simulink model "SPM_PSO"  (R2025a)
settings: Solver=VariableStepAuto  StartTime=0.0  StopTime=50000  RelTol=1e-3  AbsTol=1e-3  EnableMultiTasking=on
model workspace (MAT data in the model file):
  I = 6.58273420006
  I1 = 7.80289756193
  I2 = 6.88130880881
  SOC_break = 0.782129341538
libraries: fl_lib x8, nesl_utility x4, BatteryCurrentManagement x1, batt_lib x1, simulink x1, BatteryEstimators x1
settings Model: Creator=praji  LastModifiedBy=praji
settings SolverCC: AutoScaleAbsTol=off  AlgebraicLoopSolver=TrustRegion  MaxZcPerStep=1.0
settings DataIOCC: LimitDataPoints=on  MaxDataPoints=10000
settings OptimizationCC: ReuseModelBlockBuffer=off  LifeSpan=inf
settings DebuggingCC: UnconnectedInputMsg=warning  UnconnectedOutputMsg=warning  UnconnectedLineMsg=warning  AllowSymbolicDim=off  SFUnexpectedBacktrackingDiag=warning  SFNoUnconditionalDefaultTransitionDiag=warning  SFExecutionAtInitializationDiag=none  ArithmeticOperatorsInVariantConditions=warning
settings ModelReferenceCC: EnableRefExpFcnMdlSchedulingChecks=on
settings SFSimCC: SimUseLocalCustomCode=off  CustomCodeUndefinedFunction=UseInterfaceOnly
settings RTWCC: RTWUseLocalCustomCode=off  GPUComputeCapability=3.5  DLArmComputeVersion=19.05
settings CodeAppCC: StateflowObjectComments=on
settings GRTTargetCC: TargetLangStandard=C89/C90 (ANSI)
settings ConfigComp: CovMetricSettings=dw  CovSaveCumulativeToWorkspaceVar=on  CovSaveSingleToWorkspaceVar=on  CovExternalEMLEnable=off  CovSFcnEnable=off
settings SimscapeCC: SimscapeLogType=all  SimscapeLogSimulationStatistics=on  SimscapeLogDataHistory=10000.0

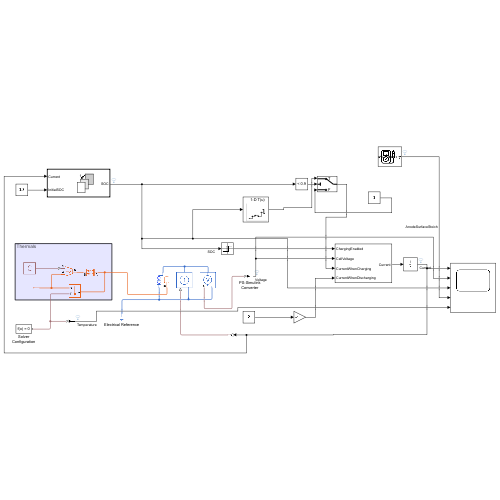
[thumbnail: Simulink's stored preview of the top-level diagram]
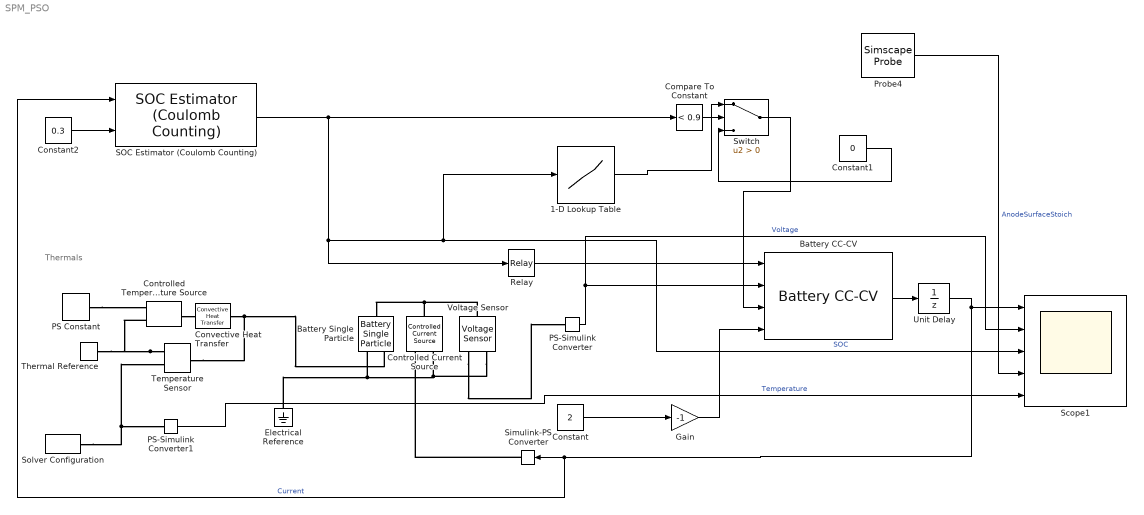
== system SPM_PSO ==
  note: Thermals
  1-D Lookup Table : Lookup_n-D  NumberOfTableDimensions=1  BreakpointsForDimension1=[0 SOC_break 1]  Table=[I1 I2 I2]  InterpMethod=Flat  InternalRulePriority=Speed  RndMeth=Simplest
  Battery CC-CV : BatteryCurrentManagement/Battery CC-CV  MinMaxFlag=off  MaxCellVoltage=3.65  Kp=100  Ki=10  Kaw=1  Kt=1  Ts=1
      settings: LibrarySourceBlock=batt_sl_lib/Current Management/Battery CC-CV
  Battery Single Particle : batt_lib/Cells/Electrochemical/Battery Single Particle  ExtrapolationMethod=simscape.enum.extrapolation.nearest  ThicknessAnode=8.52e-5 m  ElectrolyteLayerCountAnode=10  ThicknessSeparator=1.20e-5 m  ElectrolyteLayerCountSeparator=5  ThicknessCathode=7.56e-5 m  ElectrolyteLayerCountCathode=10  ElectrodePlateArea=0.177 m^2  ParticleRadiusAnode=5.86e-6 m  ShellCountAnode=20  ParticleRadiusCathode=5.22e-6 m  ShellCountCathode=25  ActiveMaterialVolumeFractionAnode=0.75  ActiveMaterialVolumeFractionCathode=0.665  StoichiometryBreakpointsSpecification=simscape.battery.enum.cells.electrochemical.StoichiometryBreakpointsSpecification.absolute  NormalizedStoichiometryBreakpoints=linspace(0.01, 0.90, 39)  OpenCircuitPotentialAnode=|  OpenCircuitPotentialCathode=|  AbsoluteStoichiometryBreakpointsAnode=linspace(0.01, 0.90, 39)  OpenCircuitPotentialAbsoluteAnode=[.484; .335; .253; .209; .2; .181; .165; .151; .139; .131; .128; .125; .124; .124; .123; .122; .119; .117; .111; .108; .101; .098; .095; .093; .092; .088; .088; .088; .088; .087; .087; .087; .085; .082; .079; .071; .064; .049; .026] V  AbsoluteStoichiometryBreakpointsCathode=linspace(0.02, 0.95, 39)  OpenCircuitPotentialAbsoluteCathode=[3.81; 3.608; 3.512; 3.478; 3.459; 3.453; 3.45257; 3.45214; 3.45171; 3.45128; 3.45085; 3.45042; 3.44999; 3.44956; 3.44913; 3.4487; 3.44827; 3.44784; 3.44741; 3.44698; 3.44655; 3.44612; 3.44569; 3.44526; 3.44483; 3.4444; 3.44397; 3.44354; 3.44311; 3.44268; 3.44225; 3.44182; 3.44139; 3.44096; 3.44053; 3.44; 3.412; 3.304; 2.968] V  MaximumConcentrationAnode=33133 mol/m^3  MaximumStoichiometryAnode=0.90  MinimumStoichiometryAnode=0.01  MaximumConcentrationCathode=63104 mol/m^3  MaximumStoichiometryCathode=0.95  MinimumStoichiometryCathode=0.02  ActiveMaterialDiffusionCoefficientAnode=3.3E-14 m^2/s  ActiveMaterialDiffusionCoefficientCathode=4E-15 m^2/s  ConductivityAnode=100 S/m  ConductivityCathode=10 S/m  CurrentCollectorResistance=0 Ohm  ElectrolyteVolumeFractionAnode=0.25  ElectrolyteVolumeFractionSeparator=0.45  ElectrolyteVolumeFractionCathode=0.335  ElectrolyteConductivity=0.29 S/m  BruggemanExponentAnode=1.5  BruggemanExponentSeparator=1.5  BruggemanExponentCathode=1.5  TransferenceNumber=0.2594  ElectrolyteDiffusionCoefficient=2.6E-10 m^2/s  ChargeTransferRateAnode=6.48e-7 m^(5/2)/(mol^(1/2)*s)  ChargeTransferRateCathode=3.42e-6 m^(5/2)/(mol^(1/2)*s)  BatteryThermalMass=50 J/K  ArrheniusReferenceTemperature=298.15 K  ActiveMaterialDiffusionActivationEnergyAnode=35000 J/mol  ActiveMaterialDiffusionActivationEnergyCathode=35000 J/mol  ElectrolyteDiffusionActivationEnergy=26600 J/mol  ConductivityActivationEnergyAnode=3000 J/mol  ConductivityActivationEnergyCathode=3000 J/mol  ElectrolyteConductivityActivationEnergy=11000 J/mol  ChargeTransferActivationEnergyAnode=35000 J/mol  ChargeTransferActivationEnergyCathode=17800 J/mol  batteryCurrent_specify=off  batteryCurrent_priority=None  batteryCurrent=0 A  batteryCurrent_nominal_specify=off  batteryCurrent_nominal_value=1  batteryCurrent_nominal_unit=A  batteryVoltage_specify=off  batteryVoltage_priority=High  batteryVoltage=3.65 V  batteryVoltage_nominal_specify=on  batteryVoltage_nominal_value=3.65  batteryVoltage_nominal_unit=V  averageElectrolyteConcentration_specify=off  averageElectrolyteConcentration_priority=High  averageElectrolyteConcentration=1200 mol/m^3  averageElectrolyteConcentration_nominal_specify=off  averageElectrolyteConcentration_nominal_value=1  averageElectrolyteConcentration_nominal_unit=mol/m^3  stateOfCharge_specify=on  stateOfCharge_priority=High  stateOfCharge=.3  stateOfCharge_nominal_specify=off  stateOfCharge_nominal_value=1  stateOfCharge_nominal_unit=1  batteryTemperature_specify=off  batteryTemperature_priority=High  batteryTemperature=298.15 K  batteryTemperature_nominal_specify=off  batteryTemperature_nominal_value=1  batteryTemperature_nominal_unit=K  power_dissipated_specify=off  power_dissipated_priority=None  power_dissipated=0 W  power_dissipated_nominal_specify=off  power_dissipated_nominal_value=1  power_dissipated_nominal_unit=W  heatGenerationRate_specify=off  heatGenerationRate_priority=None  heatGenerationRate=0 W  heatGenerationRate_nominal_specify=off  heatGenerationRate_nominal_value=1  heatGenerationRate_nominal_unit=W
      OpenCircuitPotentialAnode=|
      | [
      | 0.435; 0.325; 0.259; 0.221; 0.204; 0.194; 0.179; 0.166; 0.155;
      | 0.145; 0.137; 0.131; 0.128; 0.127; 0.126; 0.125; 0.124; 0.123;
      | 0.122; 0.121; 0.118; 0.117; 0.112; 0.109; 0.105; 0.100; 0.098;
      | 0.095; 0.094; 0.093; 0.091; 0.090; 0.089; 0.088; 0.087; 0.086;
      | 0.085; 0.084; 0.083] V
      OpenCircuitPotentialCathode=|
      | [
      | 3.598; 3.530; 3.494; 3.474; 3.460; 3.455; 3.454; 3.453; 3.4528;
      | 3.4526; 3.4524; 3.4520; 3.4518; 3.4516; 3.4514; 3.4512; 3.4510;
      | 3.4508; 3.4506; 3.4503; 3.4500; 3.4498; 3.4495; 3.4493; 3.4490;
      | 3.4488; 3.4486; 3.4484; 3.4482; 3.4479; 3.4477; 3.4475; 3.4473;
      | 3.4470; 3.4468; 3.4466; 3.4464; 3.4462; 3.4458] V
      settings: LogSimulationData=on  InternalSimscapePortConfiguration="{\"Bottom\":[],\"Left\":[{\"id\":\"p\",\"label\":\"+\",\"type\":\"foundation.electrical.electrical\"}],\"Right\":[{\"id\":\"n\",\"label\":\"-\",\"type\":\"foundation.electrical.electrical\"},{\"id\":\"H\",\"label\":\"H\",\"type\":\"foundation.thermal.thermal\"}],\"Top\":[]}"
  Compare To Constant : simulink/Logic and Bit Operations/Compare To Constant  relop=<  const=0.9  OutDataTypeStr=boolean
  Constant : Constant  Value=2
  Constant1 : Constant  Value=0
  Constant2 : Constant  Value=0.3
  Controlled Temperature Source : fl_lib/Thermal/Thermal Sources/Controlled Temperature Source
  Controlled Current Source : fl_lib/Electrical/Electrical Sources/Controlled Current Source
  Convective Heat Transfer : fl_lib/Thermal/Thermal Elements/Convective Heat Transfer  thermal_type=foundation.enum.constant_variable.constant  area=0.004 m^2  heat_tr_coeff=8 W/(K*m^2)  min_heat_tr_coeff=1e-3 W/(K*m^2)  T_specify=off  T_priority=None  T=0 K  T_nominal_specify=off  T_nominal_value=1  T_nominal_unit=K  Q_specify=off  Q_priority=None  Q=0 W  Q_nominal_specify=off  Q_nominal_value=1  Q_nominal_unit=W
  Electrical Reference : fl_lib/Electrical/Electrical Elements/Electrical Reference
  Gain : Gain  Gain=-1
  PS Constant : fl_lib/Physical Signals/Sources/PS Constant  constant=298.15 K
  PS-Simulink Converter : nesl_utility/PS-Simulink Converter  PhysicalDomain=network_engine_domain  SubClassName=ps_output  LeftPortType=input  RightPortType=output  PseudoPeriodic=off  Frequencies=[]  VectorFormat=inherit  Unit=inherit  AffineConversion=off
  PS-Simulink Converter1 : nesl_utility/PS-Simulink Converter  PhysicalDomain=network_engine_domain  SubClassName=ps_output  LeftPortType=input  RightPortType=output  PseudoPeriodic=off  Frequencies=[]  VectorFormat=inherit  Unit=inherit  AffineConversion=off
  Probe4 : SimscapeProbe  BoundBlock=28  Variables="{\"anodeModel.normalizedSurfaceStoichiometry\":{\"Probing\":\"ON\"}}"
  Relay : Relay  OnSwitchValue=0.9  OffSwitchValue=0.3  OnOutputValue=0  OffOutputValue=1
  SOC Estimator (Coulomb Counting) : BatteryEstimators/SOC Estimator (Coulomb Counting)  CurrentInputPartition=on  AH=3.4  Ts=1  DataType=Inherit: auto
      settings: LibrarySourceBlock=|
      | batt_sl_lib/Estimators/SOC Estimator
      | (Coulomb Counting)
  Scope1 : Scope  NumInputPorts=5
      settings: ActiveDisplayYMinimum=0.22431727207536242  ActiveDisplayYMaximum=0.97787657746552958
  Simulink-PS Converter : nesl_utility/Simulink-PS Converter  PhysicalDomain=network_engine_domain  SubClassName=ps_input  LeftPortType=input  RightPortType=output  PseudoPeriodic=off  Frequencies=[]  NoiseDistribution=none  NoiseParameters=[]  Unit=1  AffineConversion=off  FilteringAndDerivatives=provide  SimscapeFilterOrder=1  InputFilterTimeConstant=0.001  UdotUserProvided=0
  Solver Configuration : nesl_utility/Solver Configuration  PhysicalDomain=network_engine_domain  SubClassName=solver  LeftPortType=input  RightPortType=generic  Tones=[]  Harmonics=[]  SimulateNoise=off  Profile=off  UseLocalSampling=off  EnableSwitchedLinearOptims=on  FrequencyDomain=off  UseCCode=off  RelTol=0.001  AbsTol=1e-06  MinStep=1e-09  ToWorkspace=off  RevertToSquareIcSolve=off  NumHomotopyIterations=100  PhasorMode=off  PhasorModeNumHarmonics=1  ConsistencySolver=NEWTON_XTOL_AFTER_FTOL  IndexReductionMethod=DerivativeReplacement  DoDC=off  ResidualTolerance=1e-09  ConsistencyTolSource=GLOBAL  ConsistencyAbsTol=0.001  ConsistencyRelTol=0.001  ConsistencyTolFactor=0.001  UseLocalSolver=off  LocalSolverChoice=NE_BACKWARD_EULER_ADVANCER  ResolveIndetEquations=on  FunctionEvalNumThread=1  LocalSolverSampleTime=0.001  DoFixedCost=off  MaxNonlinIter=3  MaxModeIter=2  ComputeImpulses=off  ImpulseIterations=2  LinearAlgebra=auto  LinearAlgebraNumThread=0  EquationFormulation=NE_TIME_EF  DelaysMemoryBudget=1024  AutomaticFiltering=on  FilteringTimeConstant=0.001  PartitionStorageMethod=AS_NEEDED  PartitionMemoryBudget=1024  PartitionMethod=ROBUST  MultibodyUseLocalSolver=off  MultibodyLocalSolverChoice=ODE1  MultibodyLocalSolverSampleTime=0.001
  Switch : Switch  Criteria=u2 > Threshold  SaturateOnIntegerOverflow=off  InputSameDT=off
  Temperature Sensor : fl_lib/Thermal/Thermal Sensors/Temperature Sensor  temperature_measure=foundation.enum.MeasurementReference.difference
  Thermal Reference : fl_lib/Thermal/Thermal Elements/Thermal Reference
  Unit Delay : UnitDelay  SampleTime=-1  HasFrameUpgradeWarning=on
  Voltage Sensor : fl_lib/Electrical/Electrical Sensors/Voltage Sensor
  wires:
  PS-Simulink Converter/1 -> Scope1/2, Battery CC-CV/2  "Voltage"
  Constant/1 -> Gain/1
  SOC Estimator (Coulomb Counting)/1 -> Relay/1, 1-D Lookup Table/1, Scope1/3, Compare To Constant/1  "SOC"
  Relay/1 -> Battery CC-CV/1
  Gain/1 -> Battery CC-CV/4
  Battery CC-CV/1 -> Unit Delay/1
  Unit Delay/1 -> SOC Estimator (Coulomb Counting)/1, Simulink-PS Converter/1, Scope1/1  "Current"
  PS-Simulink Converter1/1 -> Scope1/5  "Temperature"
  1-D Lookup Table/1 -> Switch/1
  Compare To Constant/1 -> Switch/2
  Constant1/1 -> Switch/3
  Switch/1 -> Battery CC-CV/3
  Probe4/1 -> Scope1/4  "AnodeSurfaceStoich"
  Constant2/1 -> SOC Estimator (Coulomb Counting)/2
  connections:
  Electrical Reference/LConn1 -- Voltage Sensor/RConn2 -- Controlled Current Source/RConn2 -- Battery Single Particle/RConn1
  Controlled Current Source/LConn1 -- Voltage Sensor/LConn1 -- Battery Single Particle/LConn1
  Voltage Sensor/RConn1 -- PS-Simulink Converter/LConn1
  Simulink-PS Converter/RConn1 -- Controlled Current Source/RConn1
  Temperature Sensor/LConn1 -- Convective Heat Transfer/LConn1 -- Battery Single Particle/RConn2
  Temperature Sensor/RConn1 -- Thermal Reference/LConn1 -- Controlled Temperature Source/RConn2
  Controlled Temperature Source/LConn1 -- Convective Heat Transfer/RConn1
  PS Constant/RConn1 -- Controlled Temperature Source/RConn1
  Solver Configuration/RConn1 -- Temperature Sensor/RConn2 -- PS-Simulink Converter1/LConn1
